simulink model "P5_a_theta_m"  (R2024a)
settings: Solver=VariableStepAuto  StartTime=0.0  StopTime=10  RelTol=1e-3
settings Model: Creator=Rajatsurya  LastModifiedBy=Rajatsurya

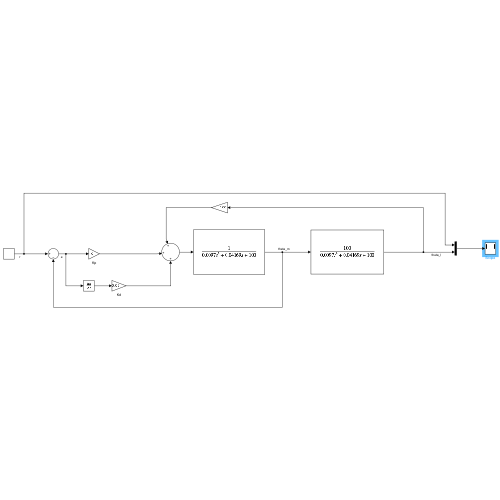
[thumbnail: Simulink's stored preview of the top-level diagram]
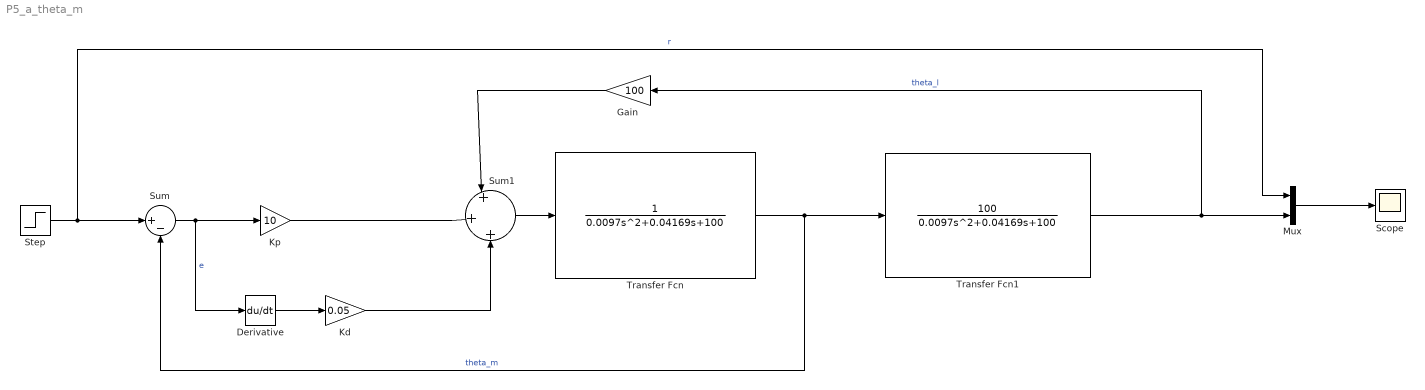
== system P5_a_theta_m ==
  Derivative : Derivative
  Gain : Gain  Gain=100
  Kd : Gain  Gain=0.05
  Kp : Gain  Gain=10
  Mux : Mux  Inputs=2
  Scope : Scope
  Step : Step  SampleTime=0
  Sum : Sum  Inputs=|+-
  Sum1 : Sum  Inputs=|+|||+|||+
  Transfer Fcn : TransferFcn  Denominator=[0.0097 0.04169 100 ]
  Transfer Fcn1 : TransferFcn  Numerator=[100]  Denominator=[0.0097 0.04169 100]
  wires:
  Step/1 -> Mux/1, Sum/1  "r"
  Sum/1 -> Derivative/1, Kp/1  "e"
  Derivative/1 -> Kd/1
  Sum1/1 -> Transfer Fcn/1
  Kp/1 -> Sum1/2
  Kd/1 -> Sum1/3
  Gain/1 -> Sum1/1
  Transfer Fcn/1 -> Sum/2, Transfer Fcn1/1  "theta_m"
  Transfer Fcn1/1 -> Mux/2, Gain/1  "theta_l"
  Mux/1 -> Scope/1
